simulink model "Controle_Digital_Aula2"  (R2022a)
settings: Solver=VariableStepAuto  StartTime=0  StopTime=10  MaxStep=1e-4  RelTol=1e-4
settings Model: Creator=luanv  LastModifiedBy=luanv

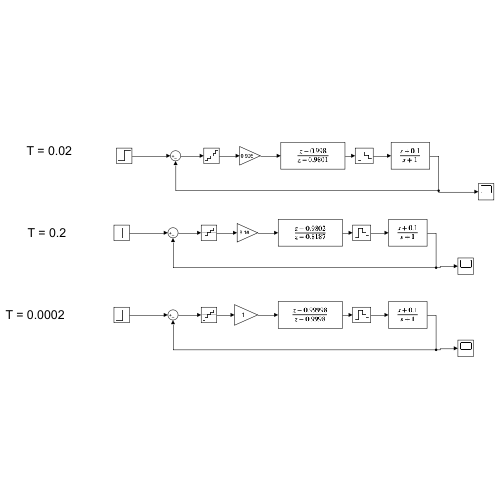
[thumbnail: Simulink's stored preview of the top-level diagram]
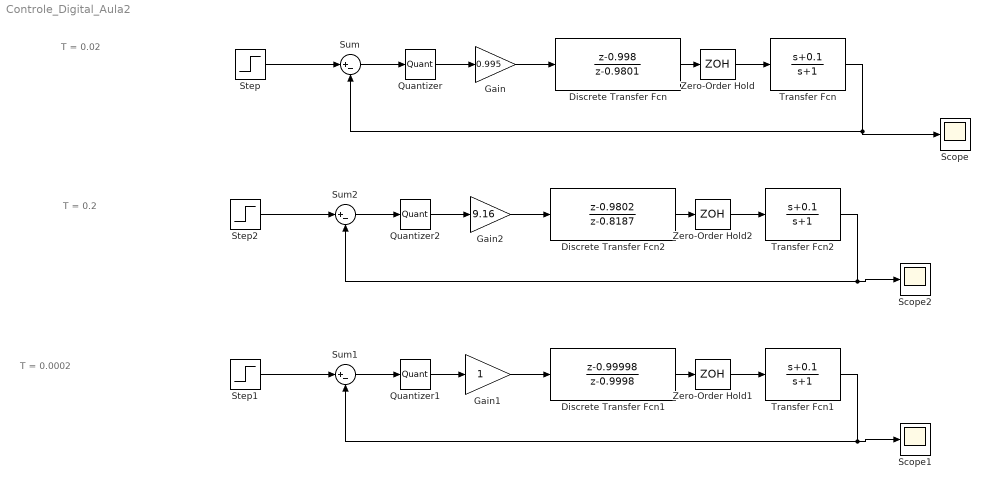
== system Controle_Digital_Aula2 ==
  note: T = 0.02
  note: T = 0.2
  note: T = 0.0002
  Discrete Transfer Fcn : DiscreteTransferFcn  Numerator=[1 -0.998]  Denominator=[1 -0.9801]
  Discrete Transfer Fcn1 : DiscreteTransferFcn  Numerator=[1 -0.99998]  Denominator=[1 -0.9998]
  Discrete Transfer Fcn2 : DiscreteTransferFcn  Numerator=[1 -0.9802]  Denominator=[1 -0.8187]
  Gain : Gain  Gain=0.995
  Gain1 : Gain
  Gain2 : Gain  Gain=9.16
  Quantizer : Quantizer  QuantizationInterval=0.0000000002
  Quantizer1 : Quantizer  QuantizationInterval=0.0000002
  Quantizer2 : Quantizer  QuantizationInterval=0.0000002
  Scope : Scope
  Scope1 : Scope
  Scope2 : Scope
  Step : Step  SampleTime=0
  Step1 : Step  SampleTime=0
  Step2 : Step  SampleTime=0
  Sum : Sum  Inputs=|+-
  Sum1 : Sum  Inputs=|+-
  Sum2 : Sum  Inputs=|+-
  Transfer Fcn : TransferFcn  Numerator=[1 0.1]  Denominator=[1 1]
  Transfer Fcn1 : TransferFcn  Numerator=[1 0.1]  Denominator=[1 1]
  Transfer Fcn2 : TransferFcn  Numerator=[1 0.1]  Denominator=[1 1]
  Zero-Order Hold : ZeroOrderHold  SampleTime=-1
  Zero-Order Hold1 : ZeroOrderHold  SampleTime=-1
  Zero-Order Hold2 : ZeroOrderHold  SampleTime=-1
  wires:
  Zero-Order Hold/1 -> Transfer Fcn/1
  Transfer Fcn/1 -> Scope/1, Sum/2
  Gain/1 -> Discrete Transfer Fcn/1
  Step/1 -> Sum/1
  Discrete Transfer Fcn/1 -> Zero-Order Hold/1
  Quantizer/1 -> Gain/1
  Sum/1 -> Quantizer/1
  Sum2/1 -> Quantizer2/1
  Transfer Fcn2/1 -> Scope2/1, Sum2/2
  Discrete Transfer Fcn2/1 -> Zero-Order Hold2/1
  Step2/1 -> Sum2/1
  Quantizer2/1 -> Gain2/1
  Gain2/1 -> Discrete Transfer Fcn2/1
  Gain1/1 -> Discrete Transfer Fcn1/1
  Quantizer1/1 -> Gain1/1
  Sum1/1 -> Quantizer1/1
  Transfer Fcn1/1 -> Scope1/1, Sum1/2
  Discrete Transfer Fcn1/1 -> Zero-Order Hold1/1
  Step1/1 -> Sum1/1
  Zero-Order Hold1/1 -> Transfer Fcn1/1
  Zero-Order Hold2/1 -> Transfer Fcn2/1
